simulink model "inc_mppt1"  (R2023a)
settings: Solver=VariableStepAuto  StartTime=0.0  StopTime=10  RelTol=1e-3
undefined symbols (not defined in the file): Acid, Lead
libraries: spsSeriesRLCBranchLib x3, spsBatteryLib x1, spsDiodeLib x1, spsMosfetLib x1, spsPVArrayLib x1, simulink x1, spspowerguiLib x1
settings Model: Creator=mluser  LastModifiedBy=mluser
settings SolverCC: ZeroCrossAlgorithm=Adaptive
settings DebuggingCC: IgnoredZcDiagnostic=none

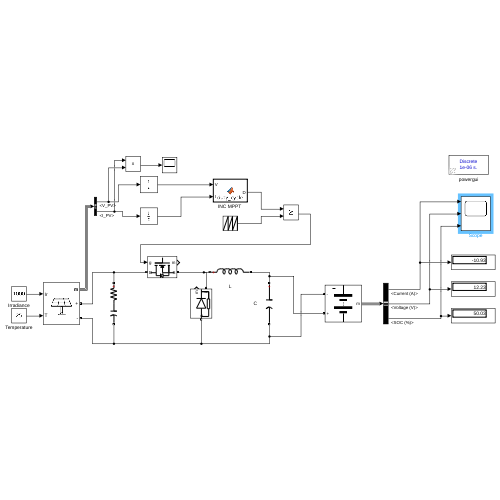
[thumbnail: Simulink's stored preview of the top-level diagram]
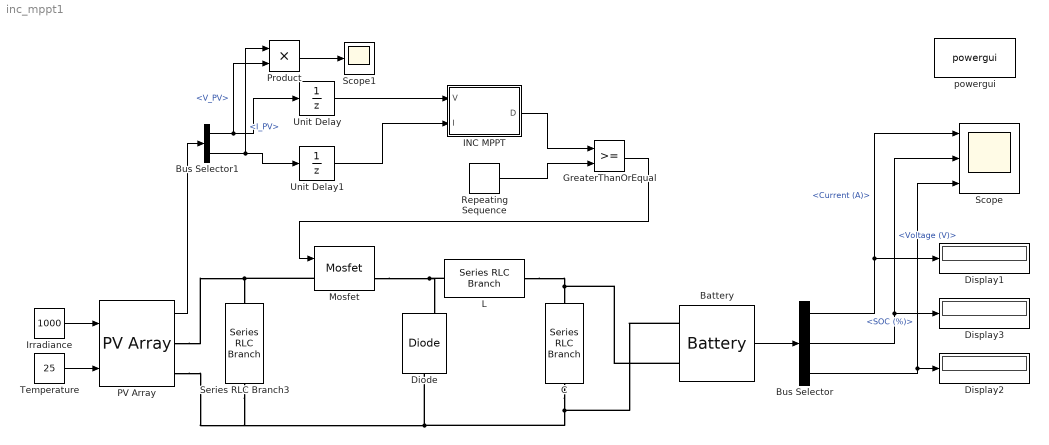
== system inc_mppt1 ==
  Battery : spsBatteryLib/Battery  BatType=Lead-Acid  ShowTempParam=off  ThermalPreset=no  ShowAgeParam=off  NomV=12  NomQ=100  SOC=50  Batt_Tr=1  PresetModel=on  MaxQ=104.1667  MinV=9  FullV=13.0658  Dis_rate=20  R=0.0012  Normal_OP=31.0278  expZone="[12.2171     0.333333]"  current=[6.5 13 32.5]  Units=Time  Tci=20  NomT=20  T2=-30  MaxQ2=4.8  FullV2=7.1  Normal_OP2=5.655  expZone2="[6.58           1]"  Rca=0.6  ti=2000  Dp=0  Neq0=0  Tsim=1e6  Ta1=25  Qeol=5.4*0.9  Reol=0.013333*1.2  Char_age=[2.3478, 3]  Dis_age=[2.3478, 10]  N1=1500  N2=10500  N3=1000  N4=1400  Ta2=45  N5=950
  Bus Selector : BusSelector  OutputSignals=Current (A),Voltage (V),SOC (%)
  Bus Selector1 : BusSelector  OutputSignals=V_PV,I_PV
  C : spsSeriesRLCBranchLib/Series RLC Branch  LConnTagsString=__new0  RConnTagsString=__new0  BranchType=C  Resistance=1  Inductance=1e-3  SetiL0=off  InitialCurrent=0  Capacitance=500e-6  Setx0=off  InitialVoltage=0  Measurements=None
  Diode : spsDiodeLib/Diode  Ron=0.001  Lon=0  Vf=0.8  IC=0  UseSnubber=0  Rs=500  Cs=250e-9  Measurements=on
  Display1 : Display
  Display2 : Display
  Display3 : Display
  GreaterThanOrEqual : RelationalOperator  OutDataTypeStr=boolean  RndMeth=Simplest  InputSameDT=off
  "INC MPPT " : MATLAB Function  TreatAsAtomicUnit=on
  Irradiance : Constant  Value=1000
  L : spsSeriesRLCBranchLib/Series RLC Branch  LConnTagsString=__new0  RConnTagsString=__new0  BranchType=L  Resistance=1  Inductance=78.125e-6  SetiL0=off  InitialCurrent=0  Capacitance=1e-6  Setx0=off  InitialVoltage=0  Measurements=None
  Mosfet : spsMosfetLib/Mosfet  Ron=0.1  Lon=0  Rd=0.01  Vfd=0  IC=0  Rs=1e5  Cs=inf  Measurements=on
  PV Array : spsPVArrayLib/PV Array  Npar=1  Nser=1  PlotType=array @ 1000 W/m2 & specified temperatures  S_vec="[ 1000  500  100 ]"  Temp_C_vec="[ 45 25  ]"  ModuleName=User-defined  PlotWhenSelected=off  Pm=441  Ncell=144  Voc=49  Isc=11  Vm=42  Im=10.5  beta_Voc_pc=-0.36099  alpha_Isc_pc=0.102  beta_Voc=-0.17689  alpha_Isc=0.01122  IL=11.0529  I0=4.0824e-10  nI=0.55149  Rsh=712.8759  Rs=0.072672  RobustModel=off  RobustCellTemperature=313.3991  BAL=on  Tc=1e-6  Tfilter=5e-5
  Product : Product
  Repeating Sequence : simulink/Sources/Repeating Sequence  rep_seq_t=[0 0.0002]  rep_seq_y=[0 1]
  Scope : Scope  NumInputPorts=3
  Scope1 : Scope
  Series RLC Branch3 : spsSeriesRLCBranchLib/Series RLC Branch  LConnTagsString=__new0  RConnTagsString=__new0  BranchType=RC  Resistance=0.001  Inductance=1e-3  SetiL0=off  InitialCurrent=0  Capacitance=0.001  Setx0=off  InitialVoltage=0  Measurements=None
  Temperature : Constant  Value=25
  Unit Delay : UnitDelay  SampleTime=-1  HasFrameUpgradeWarning=on
  Unit Delay1 : UnitDelay  SampleTime=-1  HasFrameUpgradeWarning=on
  powergui : spspowerguiLib/powergui  Priority=1  SimulationMode=Discrete  SampleTime=1e-6  frequency=60  Iterations=50  frequencyindice=0  Pbase=100e6  ErrMax=1e-4  UnitsV=kV  UnitsW=MW  buscounter=0  FunctionMessages=off  echomessages=off  EnableUseOfTLC=off  CurrentSourceSwitches=off  DisableSnubberDevices=off  DisableRonSwitches=off  DisableVfSwitches=off  DisplayEquations=off  AutomaticDiscreteSolvers=off  SolverType=Tustin/Backward Euler (TBE)  Interpol=off  ExternalGateDelay=off  methode=off  Ts=100  x0status=blocks  SPID=on  SwTol=0  HookPort=off  NonlinearTolerance=1e-4  nMaxIteration=100  ContinueOnMaxIteration=off  RestoreLinks=warning  ResistiveCurrentMeasurement=off  Frange=[0:2:500]  Ylog=off  Xlog=on  ShowGrid=off  save=off  variable=ZData  structure=0  ZoomFFT=off  StartTime=0.0  cycles=1  DisplayStyle=1  fundamental=60  FreqAxis=off  MaxFrequency=1000  frequencyindicesteady=1  RmsSteady=1  display=off
  wires:
  Battery/1 -> Bus Selector/1
  Bus Selector/2 -> Scope/2, Display3/1  "<Voltage (V)>"
  Bus Selector/3 -> Display2/1, Scope/3  "<SOC (%)>"
  Temperature/1 -> PV Array/2
  Irradiance/1 -> PV Array/1
  Bus Selector/1 -> Scope/1, Display1/1  "<Current (A)>"
  PV Array/1 -> Bus Selector1/1
  Bus Selector1/1 -> Product/2, Unit Delay/1  "<V_PV>"
  Bus Selector1/2 -> Product/1, Unit Delay1/1  "<I_PV>"
  Unit Delay/1 -> "INC MPPT "/1(V)
  Unit Delay1/1 -> "INC MPPT "/2(I)
  "INC MPPT "/1(D) -> GreaterThanOrEqual/1
  Repeating Sequence/1 -> GreaterThanOrEqual/2
  GreaterThanOrEqual/1 -> Mosfet/1
  Product/1 -> Scope1/1
  connections:
  Mosfet/RConn1 -- Diode/RConn1 -- L/LConn1
  Battery/LConn2 -- Series RLC Branch3/RConn1 -- PV Array/RConn2 -- Diode/LConn1 -- C/RConn1
  L/RConn1 -- Battery/LConn1 -- C/LConn1
  Mosfet/LConn1 -- PV Array/RConn1 -- Series RLC Branch3/LConn1

== matlab function inc_mppt1/INC MPPT  ==
  data: V input; D output; I input
function D = duty_cycle(V, I)
Dmax = 0.95;
Dmin =0;

Di =  0.95;
DelD = 0.001;
persistent   Pprev Vprev Dprev ;
if isempty(Vprev)
  Vprev = 0;
  Pprev = 0;
  Dprev = Di;
end

P= V*I;
dV=V - Vprev;
dP = P - Pprev;
if dP ~= 0
    if dP < 0
        if  dV < 0
            D =Dprev + DelD;
        else
            D = Dprev -  DelD; 
            end
    else
        if dV >0
            D = Dprev+DelD;      
        else
            D = Dprev - DelD;
        end
    end
else D = Dprev
end 

if D>= Dmax|| D< Dmin
    D= Dprev;

end

P= Pprev;
V=Vprev;
D= Dprev;
